simulink model "mil_testing_model2"  (R2022b)
settings: Solver=FixedStepDiscrete  StartTime=0.0  StopTime=7  FixedStep=1  RelTol=1e-3
undefined symbols (not defined in the file or in its folder): sigbuilder_block
settings Model: Creator=Brigosha_Guest  LastModifiedBy=Brigosha_Guest
settings ConfigComp: CovMetricSettings=dcmwe

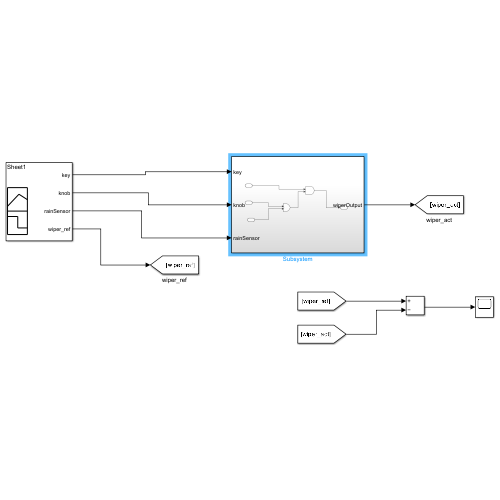
[thumbnail: Simulink's stored preview of the top-level diagram]
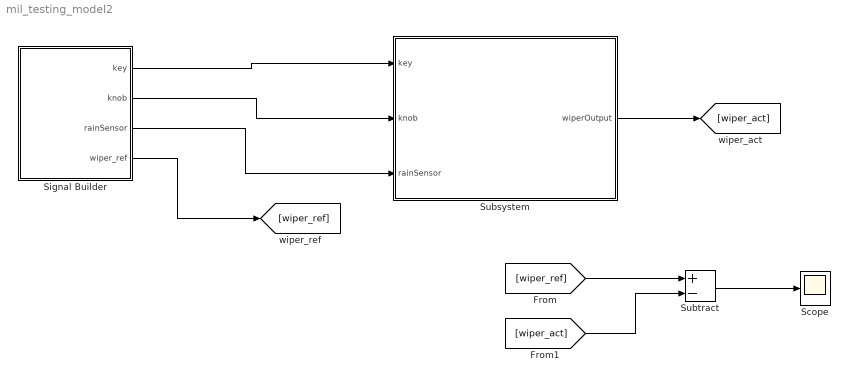
== system mil_testing_model2 ==
  Scope : Scope
  Signal Builder : Subsystem  Tag=STV Subsys  LoadFcn=sigbuilder_block('load');  StartFcn=sigbuilder_block('start');  StopFcn=sigbuilder_block('stop');  ClipboardFcn=sigbuilder_block('clipboard');  mask(Sigbuilder block){tuvar=[0:10]}
      mask help: Simulink:masks:SigbuilderBlock_MD
      mask init:
      | if ~strcmp(get_param(bdroot(gcbh),'SimulationStatus'),'stopped') tuvar = sigbuilder_block('maskInit'); end
      settings: CopyFcn=sigbuilder_block('copy');  DeleteFcn=sigbuilder_block('delete');  ModelCloseFcn=sigbuilder_block('modelClose');  PreSaveFcn=sigbuilder_block('preSave');  PauseFcn=sigbuilder_block('pause');  ContinueFcn=sigbuilder_block('continue');  NameChangeFcn=sigbuilder_block('namechange');  OpenFcn=sigbuilder_block('open',[183 81.75 550.5 359.25 ]);  CloseFcn=sigbuilder_block('close');
      mask Display: plot(0, 0, 100, 100,[2, 2, 32, 32, 2], [68, 8, 8, 68, 68],[32, 2], [38, 38], [32, 19, 2],[53, 60, 44], [32, 17, 17, 2],[16, 16, 31, 31]);txt = getActiveGroup(gcbh);text(2, 100, txt,'verticalAlignment', 'top');
  Subsystem : Subsystem
  Subtract : Sum  Inputs=+-
  wires:
  [wiper_act] -> Subtract/2
  Subtract/1 -> Scope/1
  [wiper_ref] -> Subtract/1
  Signal Builder/2(knob) -> Subsystem/2(knob)
  Signal Builder/1(key) -> Subsystem/1(key)
  Subsystem/1(wiperOutput) -> [wiper_act]
  Signal Builder/3(rainSensor) -> Subsystem/3(rainSensor)
  Signal Builder/4(wiper_ref) -> [wiper_ref]

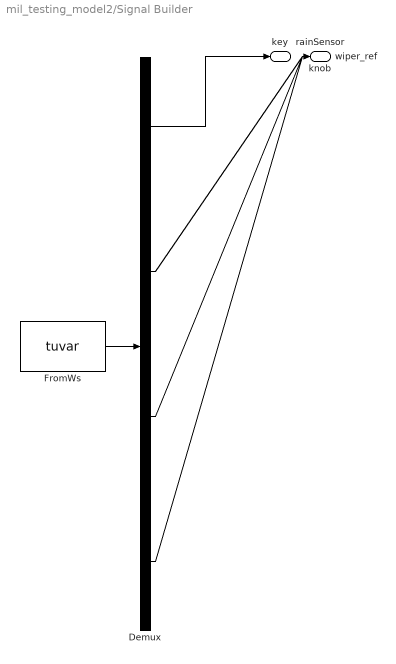
== system mil_testing_model2/Signal Builder ==
  Demux : Demux  Tag=STV Demux
      settings: DisplayOption=none
  FromWs : FromWorkspace  Tag=STV FromWs  VariableName=tuvar
      SigBuilderData=|
      | common.afterFinalStr = 'Extrapolate'
      | common.sampleTime = 0
      | dataSet.timeRange = [0 7]
      | dataSet.name = 'Sheet1'
      | sbobj.Name = 'Signal Builder'
      | sbobj.Groups.Name = 'Sheet1'
      | sbobj.Groups.Signals(1).Name = 'key'
      | sbobj.Groups.Signals(1).XData = [0 1 2 3 4 5 6 7]
      | sbobj.Groups.Signals(1).YData = [0 1 1 1 1 0 0 0]
      | sbobj.Groups.Signals(2).Name = 'knob'
      | sbobj.Groups.Signals(2).XData = [0 1 2 3 4 5 6 7]
      | sbobj.Groups.Signals(2).YData = [0 0 1 0 1 1 1 0]
      | sbobj.Groups.Signals(3).Name = 'rainSensor'
      | sbobj.Groups.Signals(3).XData = [0 1 2 3 4 5 6 7]
      | sbobj.Groups.Signals(3).YData = [0 0 0 1 1 1 0 1]
      | sbobj.Groups.Signals(4).Name = 'wiper_ref'
      | sbobj.Groups.Signals(4).XData = [0 1 2 3 4 5 6 7]
      | sbobj.Groups.Signals(4).YData = [0 0 1 1 1 0 1 0]
      | sbobj.Groups.TimeRange = [0 7]
  key : Outport  Tag=STV Outport
  knob : Outport  Tag=STV Outport  Port=2
  rainSensor : Outport  Tag=STV Outport  Port=3
  wiper_ref : Outport  Tag=STV Outport  Port=4
  wires:
  Demux/1 -> key/1
  FromWs/1 -> Demux/1
  Demux/2 -> knob/1
  Demux/3 -> rainSensor/1
  Demux/4 -> wiper_ref/1

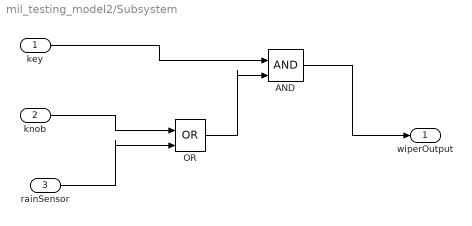
== system mil_testing_model2/Subsystem ==
  key : Inport
  knob : Inport  Port=2
  rainSensor : Inport  Port=3
  AND : Logic  IconShape=distinctive  AllPortsSameDT=off  OutDataTypeStr=boolean
  OR : Logic  Operator=OR  IconShape=distinctive  AllPortsSameDT=off  OutDataTypeStr=boolean
  wiperOutput : Outport
  wires:
  OR/1 -> AND/2
  rainSensor/1 -> OR/2
  key/1 -> AND/1
  AND/1 -> wiperOutput/1
  knob/1 -> OR/1
